simulink model "Simul_Total_Pjt"  (R2023b)
settings: Solver=FixedStepDiscrete  StartTime=0.0  StopTime=10.0  FixedStep=Ts  RelTol=1e-3
settings Model: Creator=User  LastModifiedBy=User

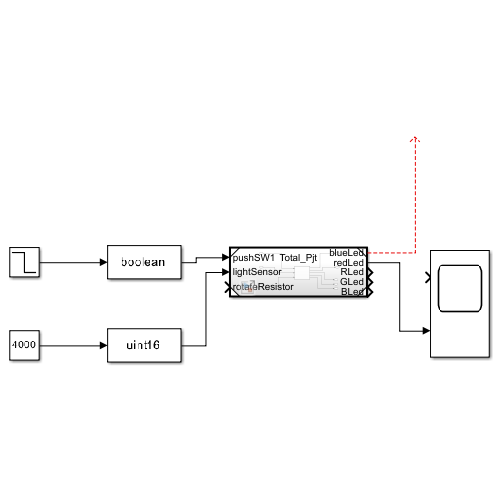
[thumbnail: Simulink's stored preview of the top-level diagram]
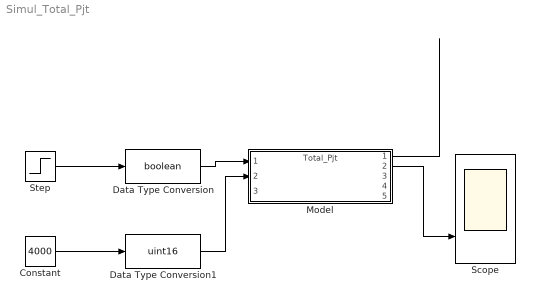
== system Simul_Total_Pjt ==
  Constant : Constant  Value=4000
  Data Type Conversion : DataTypeConversion  OutDataTypeStr=boolean  SaturateOnIntegerOverflow=off  RndMeth=Floor
  Data Type Conversion1 : DataTypeConversion  OutDataTypeStr=uint16  SaturateOnIntegerOverflow=off  RndMeth=Floor
  Model : ModelReference  ModelNameDialog=Total_Pjt.slx  SimulationMode=Normal  ModelReferenceVersion=1.9
  Scope : Scope  NumInputPorts=2
  Step : Step  Before=1  After=0  SampleTime=0
  wires:
  Step/1 -> Data Type Conversion/1
  Data Type Conversion/1 -> Model/1
  Model/1 -> ?
  Constant/1 -> Data Type Conversion1/1
  Data Type Conversion1/1 -> Model/2
  Model/2 -> Scope/2
